simulink model "sing_loop_vsg"  (R2021b)
settings: Solver=VariableStepAuto  StartTime=0.0  StopTime=10.0  RelTol=1e-3
values from neighbouring files (symbols this model uses):
  Cf_1 = 16e-6    (= 1.6e-05)    [parameters.m]
  G_int = c2d(tf([wv 0],[1 wv]),Ts/2,'tustin')    [parameters.m]
  Lf_1 = 5.6e-3    (= 0.0056)    [parameters.m]
  Lv = kQ/wn    [parameters.m]
  Pr = 2000    [parameters.m]
  RCf_1 = 0    [parameters.m]
  Rf_1 = 0.1    [parameters.m]
  Rv = kQ/10    [parameters.m]
  Ts = 1/fs    (= 0.0003125)    [parameters.m]
  Ts_sim = Ts/100    (= 3.125e-06)    [parameters.m]
  Vdc = 800*sf_v    [parameters.m]
  Vn = 181*sqrt(2)*sf_v    [parameters.m]
  wn = 2*pi*fn    (= 314.159265359)    [parameters.m]
undefined symbols (not defined in the file or in its folder): DiscIntNeverNeededParam
libraries: spsVoltageMeasurementLib x9, spsabctoAlphaBetaZeroLib x9, spsCurrentMeasurementLib x6, eeGeneralControl x5, spsThreePhaseSeriesRLCBranchLib x4, spsThreePhaseVIMeasurementLib x2, spsGroundLib x2, spsabctodq0Lib x2, spsThreePhaseSourceLib x1, eePMU x1, spsDCVoltageSourceLib x1, spsAlphaBetaZerotoabcLib x1
settings Model: Creator=Thanh Hung Mai  LastModifiedBy=Thanh Hung Mai
settings DebuggingCC: UnconnectedInputMsg=none  UnconnectedOutputMsg=none  UnconnectedLineMsg=none
settings ModelReferenceCC: EnableRefExpFcnMdlSchedulingChecks=off
settings RTWCC: DLArmComputeVersion=20.02.1

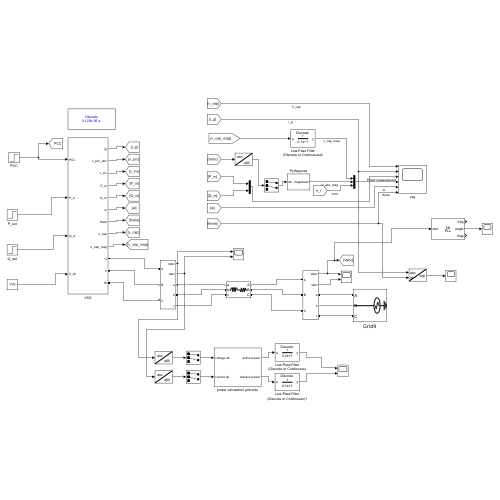
[thumbnail: Simulink's stored preview of the top-level diagram]
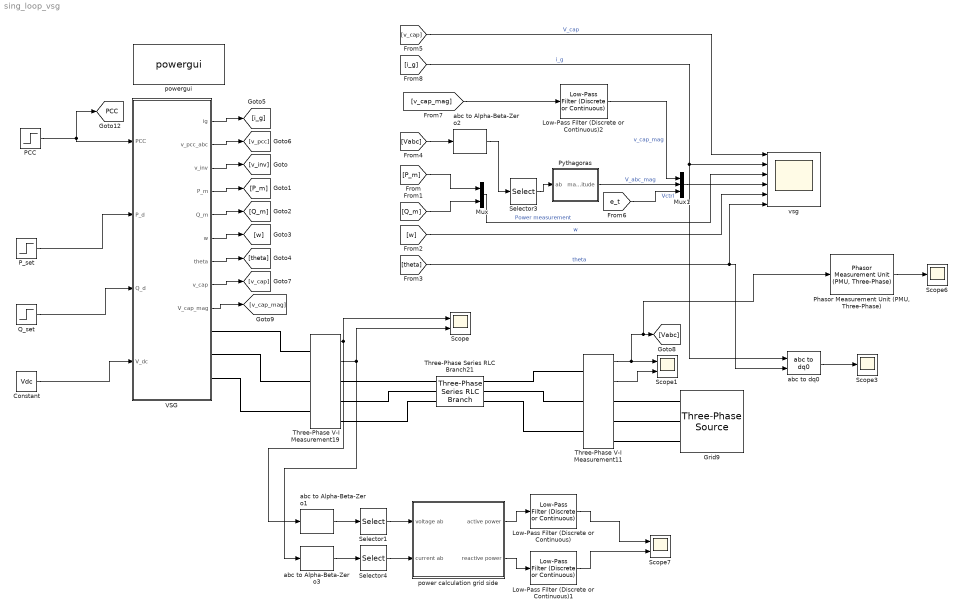
== system sing_loop_vsg ==
  Constant : Constant  Value=Vdc
  Grid9 : spsThreePhaseSourceLib/Three-Phase Source  InternalConnection=Yg  VoltagePhases=off  Voltage=sqrt(3)*Vn/(sqrt(2))  PhaseAngle=0  Voltage_phases=[25e3 25e3 25e3]/sqrt(3)  PhaseAngles_phases=[0 -120 +120]  Frequency=50*1.00  NonIdealSource=off  SpecifyImpedance=off  Resistance=0  Inductance=0  ShortCircuitLevel=10e6  BaseVoltage=sqrt(3)*Vn/sqrt(2)  XRratio=2  BusType=swing  Pref=0  Qref=0  Prefabc=[10e3, 10e3, 10e3]  Qrefabc=[0, 0, 0]  Qmin=-inf  Qmax=inf
  Low-Pass Filter (Discrete or Continuous) : eeGeneralControl/Low-Pass Filter (Discrete or Continuous)  K=1  T=0.2  B=inf  A=-inf  init_option=Inherited from block input  x0=0  Ts=-1
  Low-Pass Filter (Discrete or Continuous)1 : eeGeneralControl/Low-Pass Filter (Discrete or Continuous)  K=1  T=0.1  B=inf  A=-inf  init_option=Inherited from block input  x0=0  Ts=-1
  Low-Pass Filter (Discrete or Continuous)2 : eeGeneralControl/Low-Pass Filter (Discrete or Continuous)  K=1  T=0.1  B=inf  A=-inf  init_option=Inherited from block input  x0=0  Ts=-1
  Mux : Mux  Inputs=2
  Mux1 : Mux  Inputs=3
  PCC : Step  Time=0.5  SampleTime=Ts_sim
  P_set : Step  After=1500  SampleTime=Ts_sim
  "Phasor Measurement Unit (PMU, Three-Phase)" : eePMU/Phasor Measurement Unit (PMU, Three-Phase)  frequency=50  Nsr=48  k=1
  Pythagoras : Subsystem
  Q_set : Step  Time=5  After=0  SampleTime=Ts_sim
  Scope : Scope  NumInputPorts=2
  Scope1 : Scope  NumInputPorts=2
  Scope3 : Scope
  Scope6 : Scope
  Scope7 : Scope  NumInputPorts=2
  Selector1 : Selector  IndexMode=Zero-based  InputPortWidth=3  IndexOptions=Index vector (dialog)  Indices=[0 1]  OutputSizes=1
  Selector3 : Selector  IndexMode=Zero-based  InputPortWidth=3  IndexOptions=Index vector (dialog)  Indices=[0 1]  OutputSizes=1
  Selector4 : Selector  IndexMode=Zero-based  InputPortWidth=3  IndexOptions=Index vector (dialog)  Indices=[0 1]  OutputSizes=1
  Three-Phase Series RLC Branch21 : spsThreePhaseSeriesRLCBranchLib/Three-Phase Series RLC Branch  LConnTagsString=A|B|C  RConnTagsString=A|B|C  BranchType=RL  Resistance=0.55  Inductance=4.39e-3  Capacitance=1e-6  Measurements=None
  Three-Phase V-I Measurement11 : spsThreePhaseVIMeasurementLib/Three-Phase V-I Measurement  VoltageMeasurement=phase-to-ground  SetLabelV=off  LabelV=Vabc  Vpu=off  VpuLL=off  CurrentMeasurement=yes  SetLabelI=off  LabelI=Iabc  Ipu=off  Pbase=100e6  Vbase=500e3  OutputType=Complex  PhasorSimulation=off  PSBequivalent=0
  Three-Phase V-I Measurement19 : spsThreePhaseVIMeasurementLib/Three-Phase V-I Measurement  VoltageMeasurement=phase-to-ground  SetLabelV=off  LabelV=Vabc  Vpu=off  VpuLL=off  CurrentMeasurement=yes  SetLabelI=off  LabelI=Iabc  Ipu=off  Pbase=100e6  Vbase=500e3  OutputType=Complex  PhasorSimulation=off  PSBequivalent=0
  VSG : Subsystem  VariantControl=cascaded
  abc to Alpha-Beta-Zero1 : spsabctoAlphaBetaZeroLib/abc to Alpha-Beta-Zero
  abc to Alpha-Beta-Zero2 : spsabctoAlphaBetaZeroLib/abc to Alpha-Beta-Zero
  abc to Alpha-Beta-Zero3 : spsabctoAlphaBetaZeroLib/abc to Alpha-Beta-Zero
  abc to dq0 : spsabctodq0Lib/abc to dq0  Alignment=90 degrees behind phase A axis
  power calculation grid side : Subsystem
  powergui : spspowerguiLib/powergui  Priority=1  SimulationMode=Discrete  SampleTime=Ts_sim  frequency=60  Iterations=50  frequencyindice=0  Pbase=100e6  ErrMax=1e-4  UnitsV=kV  UnitsW=MW  buscounter=0  FunctionMessages=off  echomessages=off  EnableUseOfTLC=off  CurrentSourceSwitches=off  DisableSnubberDevices=off  DisableRonSwitches=off  DisableVfSwitches=off  DisplayEquations=off  AutomaticDiscreteSolvers=off  SolverType=Backward Euler  Interpol=off  ExternalGateDelay=off  methode=off  Ts=0  x0status=blocks  SPID=on  SwTol=0  HookPort=off  NonlinearTolerance=1e-4  nMaxIteration=100  ContinueOnMaxIteration=off  RestoreLinks=warning  ResistiveCurrentMeasurement=off  Frange=[0:2:500]  Ylog=off  Xlog=on  ShowGrid=off  save=off  variable=ZData  structure=0  ZoomFFT=off  StartTime=0.0  cycles=1  DisplayStyle=1  fundamental=60  FreqAxis=off  MaxFrequency=1000  frequencyindicesteady=1  RmsSteady=1  display=off
  vsg : Scope  NumInputPorts=6
  tag scope: PCC=global
  wires:
  [v_cap_mag] -> Low-Pass Filter (Discrete or Continuous)2/1
  Three-Phase V-I Measurement19/1 -> abc to Alpha-Beta-Zero1/1, Scope/1
  [e_t] -> Mux1/3  "Vctrl"
  VSG/6(w) -> [w]
  PCC/1 -> VSG/1(PCC), [PCC]
  power calculation grid side/2(reactive power) -> Low-Pass Filter (Discrete or Continuous)1/1
  [P_m] -> Mux/1
  [i_g] -> abc to dq0/1, vsg/2  "i_g"
  abc to dq0/1 -> Scope3/1
  Selector3/1 -> Pythagoras/1(ab)
  [Vabc] -> abc to Alpha-Beta-Zero2/1
  [v_cap] -> vsg/1  "V_cap"
  [Q_m] -> Mux/2
  [w] -> vsg/5  "w"
  abc to Alpha-Beta-Zero1/1 -> Selector1/1
  Selector1/1 -> power calculation grid side/1(voltage ab)
  Selector4/1 -> power calculation grid side/2(current ab)
  "Phasor Measurement Unit (PMU, Three-Phase)"/2 -> Scope6/1
  power calculation grid side/1(active power) -> Low-Pass Filter (Discrete or Continuous)/1
  abc to Alpha-Beta-Zero3/1 -> Selector4/1
  Q_set/1 -> VSG/3(Q_d)
  VSG/1(ig) -> [i_g]
  Three-Phase V-I Measurement11/1 -> "Phasor Measurement Unit (PMU, Three-Phase)"/1, [Vabc], Scope1/1
  Mux/1 -> vsg/3  "Power measurement"
  Low-Pass Filter (Discrete or Continuous)1/1 -> Scope7/2
  VSG/3(v_inv) -> [v_inv]
  Constant/1 -> VSG/4(V_dc)
  Three-Phase V-I Measurement11/2 -> Scope1/2
  Three-Phase V-I Measurement19/2 -> abc to Alpha-Beta-Zero3/1, Scope/2
  VSG/9(V_cap_mag) -> [v_cap_mag]
  Low-Pass Filter (Discrete or Continuous)2/1 -> Mux1/1  "v_cap_mag"
  Low-Pass Filter (Discrete or Continuous)/1 -> Scope7/1
  abc to Alpha-Beta-Zero2/1 -> Selector3/1
  [theta] -> abc to dq0/2, vsg/6  "theta"
  Mux1/1 -> vsg/4
  VSG/4(P_m) -> [P_m]
  VSG/2(v_pcc_abc) -> [v_pcc]
  VSG/7(theta) -> [theta]
  VSG/8(v_cap) -> [v_cap]
  VSG/5(Q_m) -> [Q_m]
  P_set/1 -> VSG/2(P_d)
  Pythagoras/1(magnitude) -> Mux1/2  "V_abc_mag"
  connections:
  Three-Phase V-I Measurement11/RConn1 -- Grid9/RConn1
  VSG/RConn1 -- Three-Phase V-I Measurement19/LConn1
  Three-Phase Series RLC Branch21/RConn3 -- Three-Phase V-I Measurement19/RConn3
  Three-Phase V-I Measurement11/RConn3 -- Grid9/RConn3
  Three-Phase Series RLC Branch21/LConn3 -- Three-Phase V-I Measurement11/LConn3
  Three-Phase Series RLC Branch21/RConn2 -- Three-Phase V-I Measurement19/RConn2
  Grid9/RConn2 -- Three-Phase V-I Measurement11/RConn2
  Three-Phase V-I Measurement11/LConn1 -- Three-Phase Series RLC Branch21/LConn1
  Three-Phase Series RLC Branch21/LConn2 -- Three-Phase V-I Measurement11/LConn2
  VSG/RConn2 -- Three-Phase V-I Measurement19/LConn2
  VSG/RConn3 -- Three-Phase V-I Measurement19/LConn3
  Three-Phase Series RLC Branch21/RConn1 -- Three-Phase V-I Measurement19/RConn1

== system sing_loop_vsg/Pythagoras ==
  ab : Inport
  Sqrt : Sqrt  SaturateOnIntegerOverflow=on
  Square : Math  Operator=square  SignedPower=on  RndMeth=Zero  SaturateOnIntegerOverflow=on
  Sum of Elements : Sum  Inputs=+
  magnitude : Outport  VectorParamsAs1DForOutWhenUnconnected=off
  wires:
  Sqrt/1 -> magnitude/1
  ab/1 -> Square/1
  Square/1 -> Sum of Elements/1
  Sum of Elements/1 -> Sqrt/1

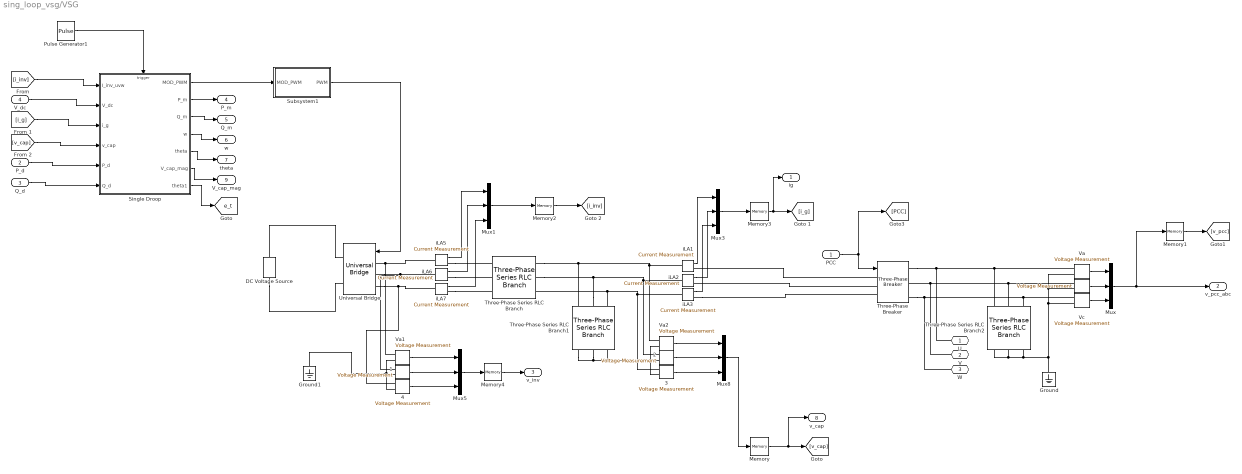
== system sing_loop_vsg/VSG ==
  PCC : Inport
  P_d : Inport  Port=2
  Q_d : Inport  Port=3
  V_dc : Inport  Port=4
     {,1..4} (5 alike) : spsVoltageMeasurementLib/Voltage Measurement  PhasorSimulation=off  OutputType=Complex  PSBequivalent=0
  DC Voltage Source : spsDCVoltageSourceLib/DC Voltage Source  Amplitude=Vdc  Measurements=None
  Ground : spsGroundLib/Ground  LConnTagsString=a
  Ground1 : spsGroundLib/Ground  LConnTagsString=a
  Memory{,1..4} (5 alike) : Memory
  Mux{,1,3,5,8} (5 alike) : Mux  Inputs=3
  Pulse Generator1 : DiscretePulseGenerator  PulseType=Time based  Period=Ts/2%1/1.5e5  PulseWidth=50
  Single Droop : Subsystem
  Subsystem1 : Subsystem
  Three-Phase Series RLC Branch : spsThreePhaseSeriesRLCBranchLib/Three-Phase Series RLC Branch  LConnTagsString=A|B|C  RConnTagsString=A|B|C  BranchType=RL  Resistance=Rf_1  Inductance=Lf_1  Capacitance=1e-6  Measurements=None
  Three-Phase Series RLC Branch1 : spsThreePhaseSeriesRLCBranchLib/Three-Phase Series RLC Branch  LConnTagsString=A|B|C  RConnTagsString=A|B|C  BranchType=RC  Resistance=RCf_1  Inductance=0.1e-3  Capacitance=Cf_1  Measurements=None
  Three-Phase Series RLC Branch2 : spsThreePhaseSeriesRLCBranchLib/Three-Phase Series RLC Branch  LConnTagsString=A|B|C  RConnTagsString=A|B|C  BranchType=R  Resistance=400e3  Inductance=0.1e-3  Capacitance=Cf_1  Measurements=None
  Three-Phase Breaker : spsThreePhaseBreakerLib/Three-Phase Breaker  InitialState=open  SwitchA=on  SwitchB=on  SwitchC=on  SwitchTimes=[0.1 0.9]  External=on  BreakerResistance=Ronb  SnubberResistance=Rsb  SnubberCapacitance=inf  Measurements=None
  Universal Bridge : spsUniversalBridgeLib/Universal Bridge  Arms=3  SnubberResistance=Rsi  SnubberCapacitance=inf  Device=IGBT / Diodes  Ron=Roni  Lon=0  ForwardVoltages="[  0  0  ]"  ForwardVoltage=0  GTOparameters=[ 10e-6 , 20e-6 ]  IGBTparameters=[ 1e-6 , 2e-6 ]  Measurements=None  Measurements_2=None  converterType=Rectifier
  Va : spsVoltageMeasurementLib/Voltage Measurement  PhasorSimulation=off  OutputType=Complex  PSBequivalent=0
  Va1 : spsVoltageMeasurementLib/Voltage Measurement  PhasorSimulation=off  OutputType=Complex  PSBequivalent=0
  Va2 : spsVoltageMeasurementLib/Voltage Measurement  PhasorSimulation=off  OutputType=Complex  PSBequivalent=0
  Vc : spsVoltageMeasurementLib/Voltage Measurement  PhasorSimulation=off  OutputType=Complex  PSBequivalent=0
  iLA{1..3,5..7} (6 alike) : spsCurrentMeasurementLib/Current Measurement  PhasorSimulation=off  OutputType=Complex  PSBequivalent=0
  U : PMIOPort  Side=Right
  V : PMIOPort  Port=2  Side=Right
  W : PMIOPort  Port=3  Side=Right
  ig : Outport  VectorParamsAs1DForOutWhenUnconnected=off
  v_pcc_abc : Outport  Port=2  VectorParamsAs1DForOutWhenUnconnected=off
  v_inv : Outport  Port=3  VectorParamsAs1DForOutWhenUnconnected=off
  P_m : Outport  Port=4
  Q_m : Outport  Port=5
  w : Outport  Port=6
  theta : Outport  Port=7
  v_cap : Outport  Port=8  VectorParamsAs1DForOutWhenUnconnected=off
  V_cap_mag : Outport  Port=9  VectorParamsAs1DForOutWhenUnconnected=off
  tag scope: e_t=global
  wires:
  Single Droop/1(MOD_PWM) -> Subsystem1/1(MOD_PWM)
  Mux/1 -> Memory1/1, v_pcc_abc/1
  Va2/1 -> Mux8/1
  iLA6/1 -> Mux1/2
  V_dc/1 -> Single Droop/2(V_dc)
  iLA3/1 -> Mux3/3
  PCC/1 -> [PCC], Three-Phase Breaker/1
  Va/1 -> Mux/1
  Pulse Generator1/1 -> Single Droop/Trigger
  iLA5/1 -> Mux1/1
  iLA2/1 -> Mux3/2
  iLA7/1 -> Mux1/3
  "   3"/1 -> Mux8/3
  "   "/1 -> Mux/2
  "   2"/1 -> Mux8/2
  Vc/1 -> Mux/3
  iLA1/1 -> Mux3/1
  Mux3/1 -> Memory3/1
  Subsystem1/1(PWM) -> Universal Bridge/1
  [i_g] -> Single Droop/3(i_g)
  "   4"/1 -> Mux5/3
  Va1/1 -> Mux5/1
  "   1"/1 -> Mux5/2
  Memory/1 -> v_cap/1, [v_cap]
  Memory1/1 -> [v_pcc]
  Mux1/1 -> Memory2/1
  Memory2/1 -> [i_inv]
  [i_inv] -> Single Droop/1(I_inv_uvw)
  [v_cap] -> Single Droop/4(v_cap)
  Memory3/1 -> ig/1, [i_g]
  Mux5/1 -> Memory4/1
  Memory4/1 -> v_inv/1
  Single Droop/5(theta) -> theta/1
  Single Droop/4(w) -> w/1
  Single Droop/3(Q_m) -> Q_m/1
  Single Droop/2(P_m) -> P_m/1
  Q_d/1 -> Single Droop/6(Q_d)
  P_d/1 -> Single Droop/5(P_d)
  Single Droop/6(V_cap_mag) -> V_cap_mag/1
  Mux8/1 -> Memory/1
  Single Droop/7(theta1) -> [e_t]
  connections:
  Three-Phase Series RLC Branch2/RConn2 -- "   "/LConn2 -- Va/LConn2 -- Vc/LConn2 -- Ground/LConn1 -- Three-Phase Series RLC Branch2/RConn3 -- Three-Phase Series RLC Branch2/RConn1
  iLA1/RConn1 -- Three-Phase Breaker/LConn1
  Three-Phase Breaker/RConn1 -- U/RConn1 -- Three-Phase Series RLC Branch2/LConn1 -- Va/LConn1
  DC Voltage Source/RConn1 -- Universal Bridge/RConn1
  iLA7/RConn1 -- Three-Phase Series RLC Branch/LConn3
  Va2/LConn2 -- Three-Phase Series RLC Branch1/RConn1 -- Three-Phase Series RLC Branch1/RConn2 -- Three-Phase Series RLC Branch1/RConn3 -- "   3"/LConn2 -- "   2"/LConn2
  Universal Bridge/LConn2 -- "   1"/LConn1 -- iLA6/LConn1
  iLA5/RConn1 -- Three-Phase Series RLC Branch/LConn1
  Three-Phase Series RLC Branch1/LConn2 -- Three-Phase Series RLC Branch/RConn2 -- iLA2/LConn1 -- "   2"/LConn1
  iLA6/RConn1 -- Three-Phase Series RLC Branch/LConn2
  Universal Bridge/LConn3 -- "   4"/LConn1 -- iLA7/LConn1
  iLA3/RConn1 -- Three-Phase Breaker/LConn3
  Three-Phase Series RLC Branch/RConn3 -- Three-Phase Series RLC Branch1/LConn3 -- iLA3/LConn1 -- "   3"/LConn1
  "   "/LConn1 -- Three-Phase Series RLC Branch2/LConn2 -- V/RConn1 -- Three-Phase Breaker/RConn2
  DC Voltage Source/LConn1 -- Universal Bridge/RConn2
  Universal Bridge/LConn1 -- Va1/LConn1 -- iLA5/LConn1
  iLA2/RConn1 -- Three-Phase Breaker/LConn2
  Three-Phase Series RLC Branch/RConn1 -- Three-Phase Series RLC Branch1/LConn1 -- iLA1/LConn1 -- Va2/LConn1
  Three-Phase Breaker/RConn3 -- Three-Phase Series RLC Branch2/LConn3 -- Vc/LConn1 -- W/RConn1
  Va1/LConn2 -- Ground1/LConn1 -- "   4"/LConn2 -- "   1"/LConn2

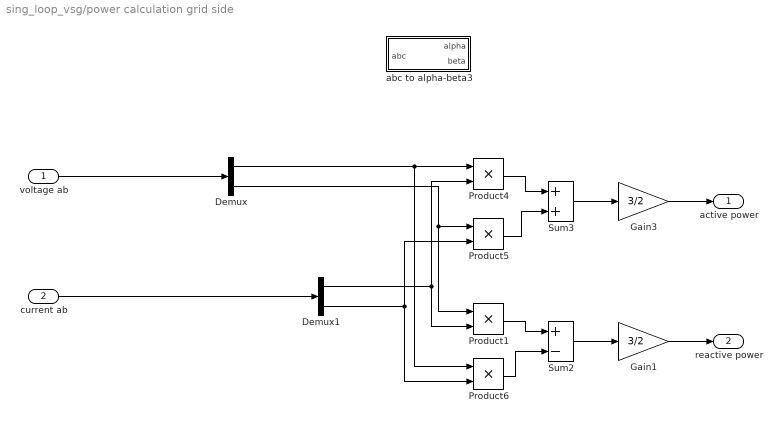
== system sing_loop_vsg/power calculation grid side ==
  voltage ab : Inport
  current ab : Inport  Port=2
  Demux : Demux  Outputs=2
  Demux1 : Demux  Outputs=2
  Gain1 : Gain  Gain=3/2
  Gain3 : Gain  Gain=3/2
  Product{1,4..6} (4 alike) : Product  InputSameDT=on  SaturateOnIntegerOverflow=on  OutDataTypeStr=Inherit: Same as first input
  Sum2 : Sum  Inputs=+-
  Sum3 : Sum
  abc to alpha-beta3 : Subsystem
  active power : Outport
  reactive power : Outport  Port=2
  wires:
  Product6/1 -> Sum2/2
  Product1/1 -> Sum2/1
  Sum2/1 -> Gain1/1
  Gain3/1 -> active power/1
  Product5/1 -> Sum3/2
  Demux1/2 -> Product5/2, Product6/2
  Demux/2 -> Product5/1, Product1/1
  Product4/1 -> Sum3/1
  Demux1/1 -> Product4/2, Product1/2
  Demux/1 -> Product6/1, Product4/1
  Sum3/1 -> Gain3/1
  Gain1/1 -> reactive power/1
  current ab/1 -> Demux1/1
  voltage ab/1 -> Demux/1

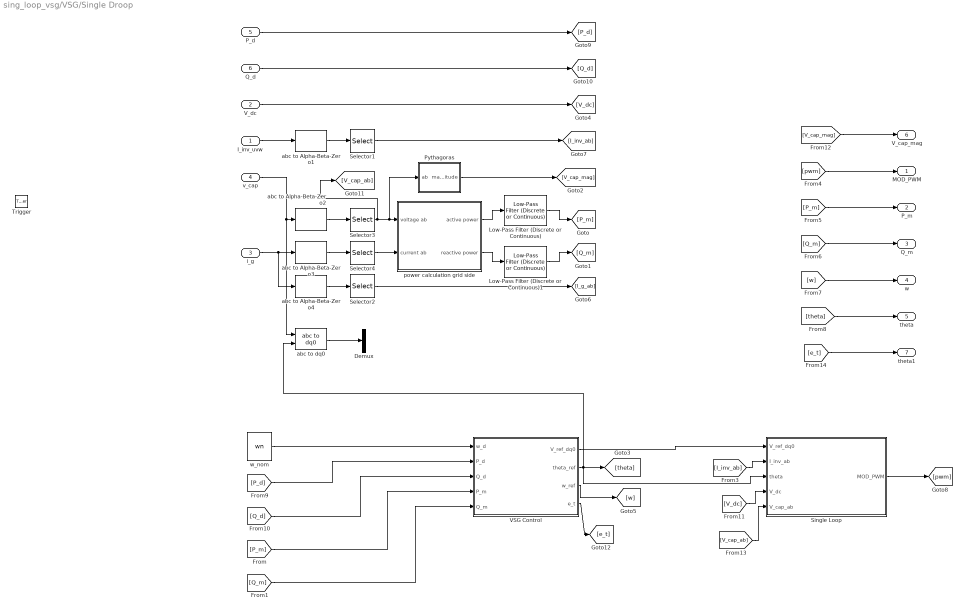
== system sing_loop_vsg/VSG/Single Droop ==
  I_inv_uvw : Inport
  V_dc : Inport  Port=2
  i_g : Inport  Port=3
  v_cap : Inport  Port=4
  P_d : Inport  Port=5
  Q_d : Inport  Port=6
  Trigger : TriggerPort  VariantControl=(inherit)  PortDimensions=1
  Demux : Demux  Outputs=3
  Low-Pass Filter (Discrete or Continuous) : eeGeneralControl/Low-Pass Filter (Discrete or Continuous)  K=1  T=0.1  B=inf  A=-inf  init_option=Inherited from block input  x0=0  Ts=-1
  Low-Pass Filter (Discrete or Continuous)1 : eeGeneralControl/Low-Pass Filter (Discrete or Continuous)  K=1  T=0.1  B=inf  A=-inf  init_option=Inherited from block input  x0=0  Ts=-1
  Pythagoras : Subsystem
  Selector{1..4} (4 alike) : Selector  IndexMode=Zero-based  InputPortWidth=3  IndexOptions=Index vector (dialog)  Indices=[0 1]  OutputSizes=1
  Single Loop : Subsystem
  VSG Control : Subsystem
  abc to Alpha-Beta-Zero{1..4} (4 alike) : spsabctoAlphaBetaZeroLib/abc to Alpha-Beta-Zero
  abc to dq0 : spsabctodq0Lib/abc to dq0  Alignment=90 degrees behind phase A axis
  power calculation grid side : Subsystem
  w_nom : Constant  Value=wn
  MOD_PWM : Outport  VectorParamsAs1DForOutWhenUnconnected=off
  P_m : Outport  Port=2  VectorParamsAs1DForOutWhenUnconnected=off
  Q_m : Outport  Port=3  VectorParamsAs1DForOutWhenUnconnected=off
  w : Outport  Port=4  VectorParamsAs1DForOutWhenUnconnected=off
  theta : Outport  Port=5  VectorParamsAs1DForOutWhenUnconnected=off
  V_cap_mag : Outport  Port=6  VectorParamsAs1DForOutWhenUnconnected=off
  theta1 : Outport  Port=7  VectorParamsAs1DForOutWhenUnconnected=off
  wires:
  abc to Alpha-Beta-Zero2/1 -> Selector3/1
  v_cap/1 -> abc to dq0/1, abc to Alpha-Beta-Zero2/1
  abc to Alpha-Beta-Zero3/1 -> Selector4/1
  i_g/1 -> abc to Alpha-Beta-Zero4/1, abc to Alpha-Beta-Zero3/1
  Pythagoras/1(magnitude) -> [V_cap_mag]
  w_nom/1 -> VSG Control/1(w_d)
  [P_d] -> VSG Control/2(P_d)
  [P_m] -> VSG Control/4(P_m)
  [Q_m] -> VSG Control/5(Q_m)
  [Q_d] -> VSG Control/3(Q_d)
  VSG Control/2(theta_ref) -> abc to dq0/2, Single Loop/3(theta), [theta]
  VSG Control/3(w_ref) -> [w]
  I_inv_uvw/1 -> abc to Alpha-Beta-Zero1/1
  abc to Alpha-Beta-Zero1/1 -> Selector1/1
  V_dc/1 -> [V_dc]
  VSG Control/1(V_ref_dq0) -> Single Loop/1(V_ref_dq0)
  abc to Alpha-Beta-Zero4/1 -> Selector2/1
  Selector2/1 -> [I_g_ab]
  [I_inv_ab] -> Single Loop/2(I_inv_ab)
  Selector1/1 -> [I_inv_ab]
  Single Loop/1(MOD_PWM) -> [pwm]
  [pwm] -> MOD_PWM/1
  [P_m] -> P_m/1
  [Q_m] -> Q_m/1
  [w] -> w/1
  [theta] -> theta/1
  P_d/1 -> [P_d]
  Q_d/1 -> [Q_d]
  [V_dc] -> Single Loop/4(V_dc)
  Selector3/1 -> [V_cap_ab], Pythagoras/1(ab), power calculation grid side/1(voltage ab)
  Selector4/1 -> power calculation grid side/2(current ab)
  power calculation grid side/1(active power) -> Low-Pass Filter (Discrete or Continuous)/1
  Low-Pass Filter (Discrete or Continuous)/1 -> [P_m]
  power calculation grid side/2(reactive power) -> Low-Pass Filter (Discrete or Continuous)1/1
  Low-Pass Filter (Discrete or Continuous)1/1 -> [Q_m]
  [V_cap_mag] -> V_cap_mag/1
  [V_cap_ab] -> Single Loop/5(V_cap_ab)
  abc to dq0/1 -> Demux/1
  VSG Control/4(e_t) -> [e_t]
  [e_t] -> theta1/1

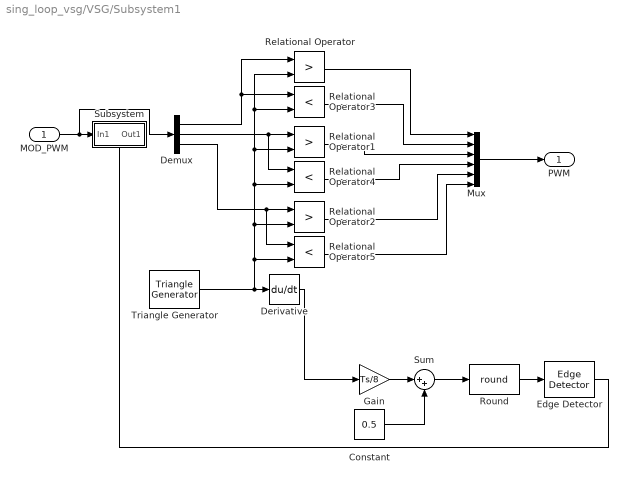
== system sing_loop_vsg/VSG/Subsystem1 ==
  MOD_PWM : Inport
  Constant : Constant  Value=0.5
  Demux : Demux  Outputs=3
  Derivative : Derivative
  Edge Detector : spsEdgeDetectorLib/Edge Detector  model=Either  ic=0  Ts=0
  Gain : Gain  Gain=Ts/8
  Mux : Mux  Inputs=6
  Relational Operator : RelationalOperator  Operator=>  OutDataTypeStr=boolean  RndMeth=Simplest
  Relational Operator1 : RelationalOperator  Operator=>  OutDataTypeStr=boolean  RndMeth=Simplest
  Relational Operator2 : RelationalOperator  Operator=>  OutDataTypeStr=boolean  RndMeth=Simplest
  Relational Operator3 : RelationalOperator  Operator=<  OutDataTypeStr=boolean  RndMeth=Simplest
  Relational Operator4 : RelationalOperator  Operator=<  OutDataTypeStr=boolean  RndMeth=Simplest
  Relational Operator5 : RelationalOperator  Operator=<  OutDataTypeStr=boolean  RndMeth=Simplest
  Round : Rounding  Operator=round
  Subsystem : Subsystem
  Sum : Sum  Inputs=|++
  Triangle Generator : spsTriangleGeneratorLib/Triangle Generator  Freq=fs  Phase=0  Ts=0
  PWM : Outport  VectorParamsAs1DForOutWhenUnconnected=off
  wires:
  Derivative/1 -> Gain/1
  Round/1 -> Edge Detector/1
  Sum/1 -> Round/1
  Constant/1 -> Sum/2
  Gain/1 -> Sum/1
  Relational Operator5/1 -> Mux/6
  Relational Operator2/1 -> Mux/5
  Relational Operator4/1 -> Mux/4
  Relational Operator1/1 -> Mux/3
  Relational Operator3/1 -> Mux/2
  Relational Operator/1 -> Mux/1
  Demux/3 -> Relational Operator2/1, Relational Operator5/1
  Demux/2 -> Relational Operator1/1, Relational Operator4/1
  Mux/1 -> PWM/1
  Demux/1 -> Relational Operator/1, Relational Operator3/1
  Triangle Generator/1 -> Relational Operator/2, Relational Operator3/2, Relational Operator1/2, Relational Operator4/2, Relational Operator2/2, Relational Operator5/2, Derivative/1
  Edge Detector/1 -> Subsystem/Trigger
  MOD_PWM/1 -> Demux/1, Subsystem/1(In1)

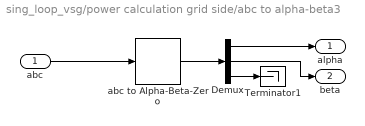
== system sing_loop_vsg/power calculation grid side/abc to alpha-beta3 ==
  abc : Inport
  Demux : Demux  Outputs=3
  Terminator1 : Terminator
  abc to Alpha-Beta-Zero : spsabctoAlphaBetaZeroLib/abc to Alpha-Beta-Zero
  alpha : Outport
  beta : Outport  Port=2
  wires:
  abc to Alpha-Beta-Zero/1 -> Demux/1
  abc/1 -> abc to Alpha-Beta-Zero/1
  Demux/3 -> Terminator1/1
  Demux/2 -> beta/1
  Demux/1 -> alpha/1

== system sing_loop_vsg/VSG/Single Droop/Pythagoras ==
  ab : Inport
  Sqrt : Sqrt  SaturateOnIntegerOverflow=on
  Square : Math  Operator=square  SignedPower=on  RndMeth=Zero  SaturateOnIntegerOverflow=on
  Sum of Elements : Sum  Inputs=+
  magnitude : Outport  VectorParamsAs1DForOutWhenUnconnected=off
  wires:
  Sqrt/1 -> magnitude/1
  ab/1 -> Square/1
  Square/1 -> Sum of Elements/1
  Sum of Elements/1 -> Sqrt/1

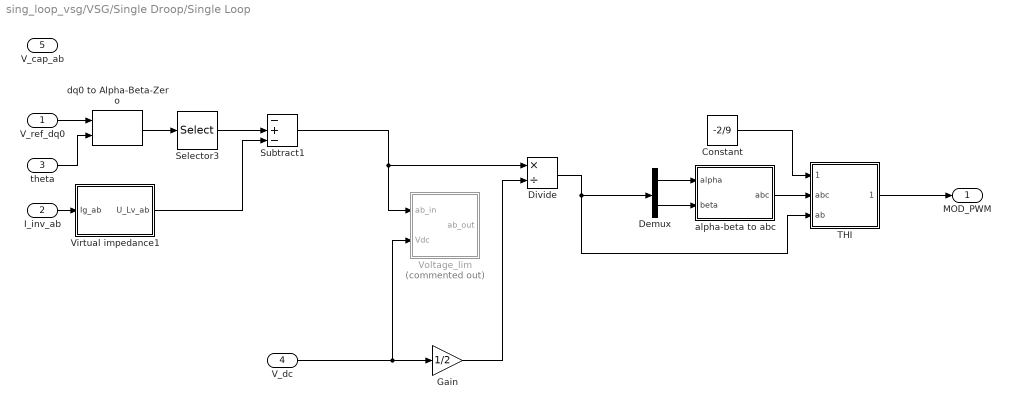
== system sing_loop_vsg/VSG/Single Droop/Single Loop ==
  V_ref_dq0 : Inport
  I_inv_ab : Inport  Port=2
  theta : Inport  Port=3
  V_dc : Inport  Port=4
  V_cap_ab : Inport  Port=5
  Constant : Constant  Value=-2/9
  Demux : Demux  Outputs=2
  Divide : Product  Inputs=*/
  Gain : Gain  Gain=1/2
  Selector3 : Selector  IndexMode=Zero-based  InputPortWidth=3  IndexOptions=Index vector (dialog)  Indices=[0 1]  OutputSizes=1
  Subtract1 : Sum  Inputs=-+-
  THI : Subsystem
  Virtual impedance1 : Subsystem
  Voltage_lim : Subsystem  Commented=on
  alpha-beta to abc : Subsystem
  dq0 to Alpha-Beta-Zero : spsdq0toAlphaBetaZeroLib/dq0 to Alpha-Beta-Zero  Alignment=90 degrees behind phase A axis
  MOD_PWM : Outport  VectorParamsAs1DForOutWhenUnconnected=off
  wires:
  Divide/1 -> Demux/1, THI/3(ab)
  V_dc/1 -> Voltage_lim/2(Vdc), Gain/1
  THI/1(abc_out) -> MOD_PWM/1
  Subtract1/1 -> Voltage_lim/1(ab_in), Divide/1
  Gain/1 -> Divide/2
  Constant/1 -> THI/1(THI gain)
  alpha-beta to abc/1(abc) -> THI/2(abc)
  I_inv_ab/1 -> Virtual impedance1/1(Ig_ab)
  Demux/1 -> alpha-beta to abc/1(alpha)
  Demux/2 -> alpha-beta to abc/2(beta)
  theta/1 -> dq0 to Alpha-Beta-Zero/2
  dq0 to Alpha-Beta-Zero/1 -> Selector3/1
  Selector3/1 -> Subtract1/2
  Virtual impedance1/1(U_Lv_ab) -> Subtract1/3
  V_ref_dq0/1 -> dq0 to Alpha-Beta-Zero/1

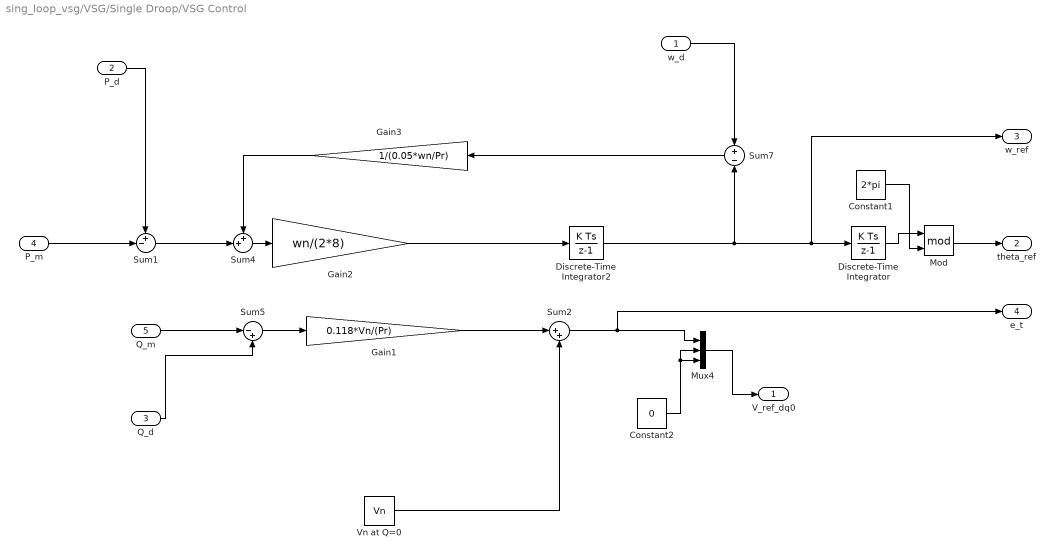
== system sing_loop_vsg/VSG/Single Droop/VSG Control ==
  w_d : Inport
  P_d : Inport  Port=2
  Q_d : Inport  Port=3
  P_m : Inport  Port=4
  Q_m : Inport  Port=5
  Constant1 : Constant  Value=2*pi
  Constant2 : Constant  Value=0
  Discrete-Time Integrator : DiscreteIntegrator  gainval=1  SampleTime=-1  ICPrevOutput=DiscIntNeverNeededParam  ICPrevScaledInput=DiscIntNeverNeededParam
  Discrete-Time Integrator2 : DiscreteIntegrator  SampleTime=-1  ICPrevOutput=DiscIntNeverNeededParam  ICPrevScaledInput=DiscIntNeverNeededParam
  Gain1 : Gain  Gain=0.118*Vn/(Pr)
  Gain2 : Gain  Gain=wn/(2*8)
  Gain3 : Gain  Gain=1/(0.05*wn/Pr)
  Mod : Math  Operator=mod  SaturateOnIntegerOverflow=on
  Mux4 : Mux  Inputs=3
  Sum1 : Sum  Inputs=+-|
  Sum2 : Sum  Inputs=|++
  Sum4 : Sum  Inputs=++|
  Sum5 : Sum  Inputs=|-+
  Sum7 : Sum  Inputs=+-
  Vn at Q=0 : Constant  Value=Vn
  V_ref_dq0 : Outport
  theta_ref : Outport  Port=2
  w_ref : Outport  Port=3
  e_t : Outport  Port=4
  wires:
  Q_m/1 -> Sum5/1
  Q_d/1 -> Sum5/2
  Vn at Q=0/1 -> Sum2/2
  Constant2/1 -> Mux4/2, Mux4/3
  Sum2/1 -> e_t/1, Mux4/1
  Mux4/1 -> V_ref_dq0/1
  Discrete-Time Integrator/1 -> Mod/1
  Mod/1 -> theta_ref/1
  Constant1/1 -> Mod/2
  Gain1/1 -> Sum2/1
  w_d/1 -> Sum7/1
  Gain2/1 -> Discrete-Time Integrator2/1
  Sum4/1 -> Gain2/1
  Discrete-Time Integrator2/1 -> Sum7/2, w_ref/1, Discrete-Time Integrator/1
  Gain3/1 -> Sum4/1
  Sum7/1 -> Gain3/1
  P_m/1 -> Sum1/2
  P_d/1 -> Sum1/1
  Sum1/1 -> Sum4/2
  Sum5/1 -> Gain1/1

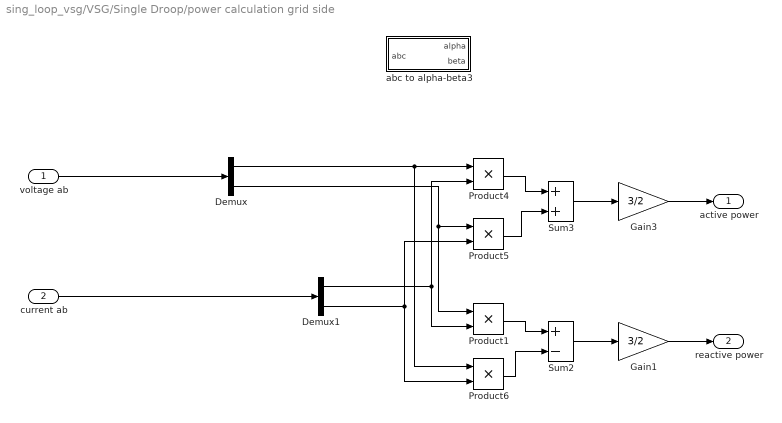
== system sing_loop_vsg/VSG/Single Droop/power calculation grid side ==
  voltage ab : Inport
  current ab : Inport  Port=2
  Demux : Demux  Outputs=2
  Demux1 : Demux  Outputs=2
  Gain1 : Gain  Gain=3/2
  Gain3 : Gain  Gain=3/2
  Product{1,4..6} (4 alike) : Product  InputSameDT=on  SaturateOnIntegerOverflow=on  OutDataTypeStr=Inherit: Same as first input
  Sum2 : Sum  Inputs=+-
  Sum3 : Sum
  abc to alpha-beta3 : Subsystem
  active power : Outport
  reactive power : Outport  Port=2
  wires:
  Product6/1 -> Sum2/2
  Product1/1 -> Sum2/1
  Sum2/1 -> Gain1/1
  Gain3/1 -> active power/1
  Product5/1 -> Sum3/2
  Demux1/2 -> Product5/2, Product6/2
  Demux/2 -> Product5/1, Product1/1
  Product4/1 -> Sum3/1
  Demux1/1 -> Product4/2, Product1/2
  Demux/1 -> Product6/1, Product4/1
  Sum3/1 -> Gain3/1
  Gain1/1 -> reactive power/1
  current ab/1 -> Demux1/1
  voltage ab/1 -> Demux/1

== system sing_loop_vsg/VSG/Subsystem1/Subsystem ==
  In1 : Inport
  Trigger : TriggerPort  VariantControl=Variant  PortDimensions=1
  Out1 : Outport  VectorParamsAs1DForOutWhenUnconnected=off
  wires:
  In1/1 -> Out1/1

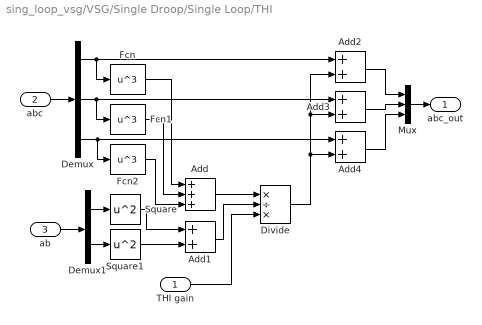
== system sing_loop_vsg/VSG/Single Droop/Single Loop/THI ==
  THI gain : Inport
  abc : Inport  Port=2
  ab : Inport  Port=3
  Add : Sum  Inputs=+++
  Add{1..4} (4 alike) : Sum
  Demux : Demux  Outputs=3
  Demux1 : Demux  Outputs=2
  Divide : Product  Inputs=*/*
  Fcn : Fcn  Expr=u^3
  Fcn1 : Fcn  Expr=u^3
  Fcn2 : Fcn  Expr=u^3
  Mux : Mux  Inputs=3
  Square : Math  Operator=square  SignedPower=on  RndMeth=Zero  SaturateOnIntegerOverflow=on
  Square1 : Math  Operator=square  SignedPower=on  RndMeth=Zero  SaturateOnIntegerOverflow=on
  abc_out : Outport  VectorParamsAs1DForOutWhenUnconnected=off
  wires:
  Demux/2 -> Add3/1, Fcn1/1
  Fcn2/1 -> Add/3
  Fcn1/1 -> Add/2
  Fcn/1 -> Add/1
  Mux/1 -> abc_out/1
  Add4/1 -> Mux/3
  Add2/1 -> Mux/1
  Add3/1 -> Mux/2
  Divide/1 -> Add4/2, Add3/2, Add2/2
  THI gain/1 -> Divide/3
  Add1/1 -> Divide/2
  Add/1 -> Divide/1
  Square1/1 -> Add1/2
  Square/1 -> Add1/1
  Demux1/2 -> Square1/1
  Demux1/1 -> Square/1
  ab/1 -> Demux1/1
  Demux/1 -> Fcn/1, Add2/1
  Demux/3 -> Add4/1, Fcn2/1
  abc/1 -> Demux/1

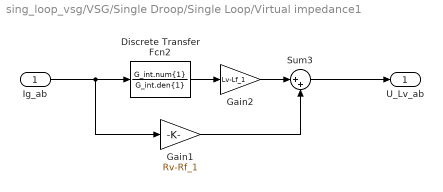
== system sing_loop_vsg/VSG/Single Droop/Single Loop/Virtual impedance1 ==
  Ig_ab : Inport
  Discrete Transfer Fcn2 : DiscreteTransferFcn  Numerator=G_int.num{1}  Denominator=G_int.den{1}
  Gain1 : Gain  Gain=Rv-Rf_1
  Gain2 : Gain  Gain=Lv-Lf_1
  Sum3 : Sum  Inputs=|++
  U_Lv_ab : Outport  VectorParamsAs1DForOutWhenUnconnected=off
  wires:
  Sum3/1 -> U_Lv_ab/1
  Gain1/1 -> Sum3/2
  Gain2/1 -> Sum3/1
  Ig_ab/1 -> Discrete Transfer Fcn2/1, Gain1/1
  Discrete Transfer Fcn2/1 -> Gain2/1

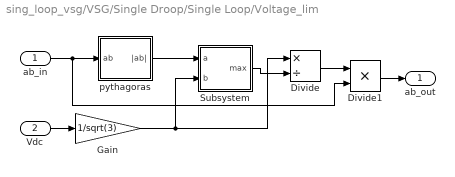
== system sing_loop_vsg/VSG/Single Droop/Single Loop/Voltage_lim ==
  ab_in : Inport
  Vdc : Inport  Port=2
  Divide : Product  Inputs=*/
  Divide1 : Product  Inputs=**
  Gain : Gain  Gain=1/sqrt(3)
  Subsystem : Subsystem
  pythagoras : Subsystem
  ab_out : Outport  VectorParamsAs1DForOutWhenUnconnected=off
  wires:
  Gain/1 -> Divide/1, Subsystem/2(b)
  ab_in/1 -> Divide1/2, pythagoras/1(ab)
  pythagoras/1(|ab|) -> Subsystem/1(a)
  Vdc/1 -> Gain/1
  Subsystem/1(max) -> Divide/2
  Divide/1 -> Divide1/1
  Divide1/1 -> ab_out/1

== system sing_loop_vsg/VSG/Single Droop/Single Loop/alpha-beta to abc ==
  alpha : Inport
  beta : Inport  Port=2
  Alpha-Beta-Zero to abc1 : spsAlphaBetaZerotoabcLib/Alpha-Beta-Zero to abc
  Constant : Constant  Value=0
  Mux1 : Mux  Inputs=3
  abc : Outport
  wires:
  alpha/1 -> Mux1/1
  Mux1/1 -> Alpha-Beta-Zero to abc1/1
  Constant/1 -> Mux1/3
  beta/1 -> Mux1/2
  Alpha-Beta-Zero to abc1/1 -> abc/1

== system sing_loop_vsg/VSG/Single Droop/power calculation grid side/abc to alpha-beta3 ==
  abc : Inport
  Demux : Demux  Outputs=3
  Terminator1 : Terminator
  abc to Alpha-Beta-Zero : spsabctoAlphaBetaZeroLib/abc to Alpha-Beta-Zero
  alpha : Outport
  beta : Outport  Port=2
  wires:
  abc to Alpha-Beta-Zero/1 -> Demux/1
  abc/1 -> abc to Alpha-Beta-Zero/1
  Demux/3 -> Terminator1/1
  Demux/2 -> beta/1
  Demux/1 -> alpha/1

== system sing_loop_vsg/VSG/Single Droop/Single Loop/Voltage_lim/Subsystem ==
  a : Inport
  b : Inport  Port=2
  Relational Operator : RelationalOperator  Operator=>  OutDataTypeStr=boolean  RndMeth=Simplest
  Switch : Switch  Criteria=u2 > Threshold  Threshold=0.5
  max : Outport  VectorParamsAs1DForOutWhenUnconnected=off
  wires:
  a/1 -> Relational Operator/1, Switch/1
  Switch/1 -> max/1
  b/1 -> Relational Operator/2, Switch/3
  Relational Operator/1 -> Switch/2

== system sing_loop_vsg/VSG/Single Droop/Single Loop/Voltage_lim/pythagoras ==
  ab : Inport
  Sqrt : Sqrt  SaturateOnIntegerOverflow=on
  Square : Math  Operator=square  SignedPower=on  RndMeth=Zero  SaturateOnIntegerOverflow=on
  Sum of Elements : Sum  Inputs=+
  |ab| : Outport  VectorParamsAs1DForOutWhenUnconnected=off
  wires:
  Sum of Elements/1 -> Sqrt/1
  ab/1 -> Square/1
  Square/1 -> Sum of Elements/1
  Sqrt/1 -> |ab|/1
